simulink library "dynamics_lib"  (R2023b)
settings: Solver=VariableStepAuto  StartTime=0.0  StopTime=10.0  RelTol=1e-3
libraries: Raptor_lib x129, cstblocks x1, autolibshared x1
(part 2 of 2)

== system dynamics_lib/vehicleModel ==
  Constant : Constant  Value=5
  Constant1 : Constant  Value=5
  Display : Display
  Scope : Scope  NumInputPorts=6
  Vehicle Body 3DOF Single Track : autolibshared/Vehicle Body 3DOF Single Track  trackMode=Single (bicycle)  inputMode=External longitudinal velocity  frontSteerMode=on  rearSteerMode=off  windMode=off  muMode=off  extFMode=off  extMMode=off  htchFMode=off  htchMMode=off  extXo=off  extpsio=off  extxdoto=off  extro=off  extYo=off  extTamb=off  extydoto=off  aMode=2  NF=2  NR=2  m=272.16  a=0.76835  b=0.76835  h=0.31612  dh=1  hh=0.2  X_o=0  xdot_o=0  CalphaMode=off  sigmaMode=off  d=0  hl=0  w=[1.4,1.4]  Cy_f=18550.11  Cy_r=18550.11  sigma_f=.1  sigma_r=.1  alpha_f_brk=[-.1 .1]  Cy_f_data=[-9e3 9e3]  alpha_r_brk=[-.1 .1]  Cy_r_data=[-9e3 9e3]  Y_o=0  ydot_o=0  Izz=113.95  psi_o=0  r_o=0  Af=1.207  Cd=.3  Cl=.1  Cpm=.1  beta_w=[0 0.01:0.01:0.3]  Cs=[0 0.01:0.01:0.3]  Cym=[0 1e-6:0.01:0.3]  Pabs=101325  Tair=273  g=9.81  mu=1  xdot_tol=.01  Fznom=5000  Fxtire_sat=7e4  Fytire_sat=7e4  longOff=0  latOff=0  vertOff=0  wrapAng=off
  wires:
  Vehicle Body 3DOF Single Track/1 -> Display/1
  Vehicle Body 3DOF Single Track/2 -> Scope/1
  Vehicle Body 3DOF Single Track/3 -> Scope/2
  Vehicle Body 3DOF Single Track/4 -> Scope/3
  Vehicle Body 3DOF Single Track/5 -> Scope/4
  Vehicle Body 3DOF Single Track/6 -> Scope/5
  Vehicle Body 3DOF Single Track/7 -> Scope/6
  Constant/1 -> Vehicle Body 3DOF Single Track/2
  Constant1/1 -> Vehicle Body 3DOF Single Track/1

== matlab function dynamics_lib/rearNSMWT/rearNSMWT ==
  data: rearNonSuspendedMass input; rearNSMWT output; MM5_ay input; rearNonSuspendedMassCGHeight input; rearTrack input
function rearNSMWT = fcn(rearNonSuspendedMass, MM5_ay, ...
    rearNonSuspendedMassCGHeight, rearTrack)

rearNSMWT = rearNonSuspendedMass*2*MM5_ay*...
    rearNonSuspendedMassCGHeight/rearTrack;

== matlab function dynamics_lib/frontGeoWT/frontGeoWT ==
  data: suspendedMass input; frontGeoWT output; suspendedMassWeightDistribution input; MM5_ay input; frontRollCenterHeight input; frontTrack input
function frontGeoWT = fcn(suspendedMass, ...
    suspendedMassWeightDistribution, MM5_ay, frontRollCenterHeight, ...
        frontTrack)

frontGeoWT = suspendedMass*(suspendedMassWeightDistribution/100)*MM5_ay*...
    frontRollCenterHeight/frontTrack;

== matlab function dynamics_lib/rearGeoWT/rearGeoWT ==
  data: suspendedMass input; rearGeoWT output; suspendedMassWeightDistribution input; MM5_ay input; rearRollCenterHeight input; rearTrack input
function rearGeoWT = fcn(suspendedMass, ...
    suspendedMassWeightDistribution, MM5_ay, rearRollCenterHeight, ...
        rearTrack)

rearGeoWT = (suspendedMass*((100-suspendedMassWeightDistribution)/100))*...
    MM5_ay*rearRollCenterHeight/rearTrack;

== matlab function dynamics_lib/antiRollFrontSprings/antiRollFrontSprings ==
  data: frontTrack input; antiRollFrontSprings output; frontWheelRate input
function antiRollFrontSprings = fcn(frontTrack, frontWheelRate)

antiRollFrontSprings = ((frontTrack/1000)^2*tan(1)* ...
    (frontWheelRate*1000))/2;

== matlab function dynamics_lib/antiRollRearSprings/antiRollRearSprings ==
  data: rearTrack input; antiRollRearSprings output; rearWheelRate input
function antiRollRearSprings = fcn(rearTrack, rearWheelRate)

antiRollRearSprings = ((rearTrack/1000)^2*tan(1)* ...
    (rearWheelRate*1000))/2;

== matlab function dynamics_lib/frontWheelRate/frontWheelRate ==
  data: frontSpringStiffness input; frontWheelRate output; frontSpringMotionRatio input
function frontWheelRate = fcn(frontSpringStiffness, frontSpringMotionRatio)

frontWheelRate = frontSpringStiffness/frontSpringMotionRatio^2;

== matlab function dynamics_lib/antiRollFrontAxleAndTire/antiRollFrontAxleAndTire ==
  data: antiRollFrontAxleAndTire output; antiRollFrontSprings input; antiRollFrontARB input; antiRollFrontTires input
function antiRollFrontAxleAndTire = fcn(antiRollFrontSprings, ...
    antiRollFrontARB, antiRollFrontTires)

antiRollFrontAxleAndTire = ((antiRollFrontSprings+antiRollFrontARB)* ...
    antiRollFrontTires)/((antiRollFrontSprings+antiRollFrontARB)+ ...
        antiRollFrontTires);

== matlab function dynamics_lib/antiRollRearAxleAndTire/antiRollRearAxleAndTire ==
  data: antiRollRearAxleAndTire output; antiRollRearSprings input; antiRollRearARB input; antiRollRearTires input
function antiRollRearAxleAndTire = fcn(antiRollRearSprings, ...
    antiRollRearARB, antiRollRearTires)

antiRollRearAxleAndTire = ((antiRollRearSprings+antiRollRearARB)* ...
    antiRollRearTires)/((antiRollRearSprings+antiRollRearARB)+ ...
        antiRollRearTires);

== matlab function dynamics_lib/antiRollTotal/antiRollTotal ==
  data: antiRollFrontAxleAndTire input; antiRollTotal output; antiRollRearAxleAndTire input
function antiRollTotal = fcn(antiRollFrontAxleAndTire, ...
    antiRollRearAxleAndTire)

antiRollTotal = antiRollFrontAxleAndTire+antiRollRearAxleAndTire;

== matlab function dynamics_lib/frontElWT/frontElWT ==
  data: frontElWT output; suspendedMass input; MM5_ay input; deltaZ input; antiRollFrontAxleAndTire input; antiRollTotal input; frontTrack input
function frontElWT = fcn(suspendedMass, MM5_ay, deltaZ, ...
    antiRollFrontAxleAndTire, antiRollTotal, frontTrack)

frontElWT = (suspendedMass*MM5_ay*deltaZ* ...
    (antiRollFrontAxleAndTire/antiRollTotal))/frontTrack;

== matlab function dynamics_lib/rearElWT/rearElWT ==
  data: rearElWT output; suspendedMass input; MM5_ay input; deltaZ input; antiRollRearAxleAndTire input; antiRollTotal input; rearTrack input
function rearElWT = fcn(suspendedMass, MM5_ay, deltaZ, ...
    antiRollRearAxleAndTire, antiRollTotal, rearTrack)

rearElWT = (suspendedMass*MM5_ay*deltaZ* ...
    (antiRollRearAxleAndTire/antiRollTotal))/rearTrack;

== matlab function dynamics_lib/frontTotalWT/frontTotalWT ==
  data: frontNSMWT input; frontTotalWT output; frontElWT input; frontGeoWT input
function frontTotalWT = fcn(frontNSMWT, frontElWT, frontGeoWT)

frontTotalWT = frontNSMWT+frontElWT+frontGeoWT;

== matlab function dynamics_lib/rearTotalWT/rearTotalWT ==
  data: rearNSMWT input; rearTotalWT output; rearElWT input; rearGeoWT input
function rearTotalWT = fcn(rearNSMWT, rearElWT, rearGeoWT)

rearTotalWT = rearNSMWT+rearElWT+rearGeoWT;

== matlab function dynamics_lib/dynamicLoadFL/dynamicLoadFL ==
  data: dynamicLoadFL output; totalMass input; totalMassDistribution input; totalDownForce input; downForceDistribution input; totalFrontWT input; gravity input
function dynamicLoadFL = fcn(totalMass, totalMassDistribution, ...
    totalDownForce, downForceDistribution, totalFrontWT, gravity)

dynamicLoadFL = (totalMass*totalMassDistribution/100*0.5+totalDownForce*...
    downForceDistribution/100/2-totalFrontWT)*gravity;

== matlab function dynamics_lib/dynamicLoadFR/dynamicLoadFR ==
  data: dynamicLoadFR output; totalMass input; totalMassDistribution input; totalDownForce input; downForceDistribution input; totalFrontWT input; gravity input
function dynamicLoadFR = fcn(totalMass, totalMassDistribution, ...
    totalDownForce, downForceDistribution, totalFrontWT, gravity)

dynamicLoadFR = (totalMass*totalMassDistribution/100*0.5+totalDownForce*...
    downForceDistribution/100/2+totalFrontWT)*gravity;

== matlab function dynamics_lib/dynamicLoadRL/dynamicLoadRL ==
  data: dynamicLoadRL output; totalMass input; totalMassDistribution input; totalDownForce input; downForceDistribution input; totalRearWT input; gravity input
function dynamicLoadRL = fcn(totalMass, totalMassDistribution, ...
    totalDownForce, downForceDistribution, totalRearWT, gravity)

dynamicLoadRL = (totalMass*(100-totalMassDistribution)/100*0.5+ ...
    totalDownForce*(100-downForceDistribution)/100/2-totalRearWT)*gravity;

== matlab function dynamics_lib/dynamicLoadRR/dynamicLoadRR ==
  data: dynamicLoadRR output; totalMass input; totalMassDistribution input; totalDownForce input; downForceDistribution input; totalRearWT input; gravity input
function dynamicLoadRR = fcn(totalMass, totalMassDistribution, ...
    totalDownForce, downForceDistribution, totalRearWT, gravity)

dynamicLoadRR = (totalMass*(100-totalMassDistribution)/100*0.5+ ...
    totalDownForce*(100-downForceDistribution)/100/2+totalRearWT)*gravity;

== matlab function dynamics_lib/fz/fz ==
  data: frontSpringStiffness input; dynamicLoadFL output; frontSpringMotionRatio input; rearSpringStiffness input; rearSpringMotionRatio input; frontNonSuspendedMass input; MM5_ay input; frontNonSuspendedMassCGHeight input; frontTrack input; suspendedMass input; suspendedMassWeightDistribution input; frontRollCenterHeight input; frontTireStiffness input; frontARBStiffness input; frontARBMotionRatio input; rearTrack input; rearARBStiffness input; rearARBMotionRatio input; rearTireStiffness input; rearNonSuspendedMass input; rearNonSuspendedMassCGHeight input; rearRollCenterHeight input; suspendedMassCGCoordinatesZ input; wheelBase input; totalMass input; totalMassDistribution input; totalDownForce input; downForceDistribution input; gravity input; dynamicLoadFR output; dynamicLoadRL output; dynamicLoadRR output
function [dynamicLoadFL, dynamicLoadFR, dynamicLoadRL, dynamicLoadRR] = ...
    fz(frontSpringStiffness, frontSpringMotionRatio, ...
    rearSpringStiffness, rearSpringMotionRatio, frontNonSuspendedMass, ...
    MM5_ay, frontNonSuspendedMassCGHeight, frontTrack, suspendedMass, ...
    suspendedMassWeightDistribution, frontRollCenterHeight, ...
    frontTireStiffness, frontARBStiffness, frontARBMotionRatio, ...
    rearTrack, rearARBStiffness, rearARBMotionRatio, ...
    rearTireStiffness, rearNonSuspendedMass, ...
    rearNonSuspendedMassCGHeight, rearRollCenterHeight, ...
    suspendedMassCGCoordinatesZ, wheelBase, totalMass, ...
    totalMassDistribution, totalDownForce, downForceDistribution, gravity)



frontWheelRate = frontSpringStiffness/frontSpringMotionRatio^2;
rearWheelRate = rearSpringStiffness/rearSpringMotionRatio^2;
frontNSMWT = frontNonSuspendedMass*2*MM5_ay*...
    frontNonSuspendedMassCGHeight/frontTrack;
frontGeoWT = suspendedMass*(suspendedMassWeightDistribution/100)*MM5_ay*...
    frontRollCenterHeight/frontTrack;
antiRollFrontTires = ((frontTrack/1000)^2*tan(1)*frontTireStiffness* ...
    1000)/2;
antiRollFrontARB = (frontARBStiffness*1000*(frontTrack/1000)^2*tan(1))/...
    frontARBMotionRatio^2;
antiRollFrontSprings = ((frontTrack/1000)^2*tan(1)* ...
    (frontWheelRate*1000))/2;
antiRollRearSprings = ((rearTrack/1000)^2*tan(1)* ...
    (rearWheelRate*1000))/2;
antiRollRearARB = (rearARBStiffness*1000*(rearTrack/1000)^2*tan(1))/...
    rearARBMotionRatio^2;
antiRollRearTires = ((rearTrack/1000)^2*tan(1)*rearTireStiffness* ...
    1000)/2;
rearNSMWT = rearNonSuspendedMass*2*MM5_ay*...
    rearNonSuspendedMassCGHeight/rearTrack;
rearGeoWT = (suspendedMass*((100-suspendedMassWeightDistribution)/100))*...
    MM5_ay*rearRollCenterHeight/rearTrack;
deltaZ = suspendedMassCGCoordinatesZ-...
    (((rearRollCenterHeight-frontRollCenterHeight)/wheelBase* ...
        ((100-suspendedMassWeightDistribution)/100*wheelBase))+ ...
            frontRollCenterHeight);
antiRollFrontAxleAndTire = ((antiRollFrontSprings+antiRollFrontARB)* ...
    antiRollFrontTires)/((antiRollFrontSprings+antiRollFrontARB)+ ...
        antiRollFrontTires);
antiRollRearAxleAndTire = ((antiRollRearSprings+antiRollRearARB)* ...
    antiRollRearTires)/((antiRollRearSprings+antiRollRearARB)+ ...
        antiRollRearTires);
antiRollTotal = antiRollFrontAxleAndTire+antiRollRearAxleAndTire;
frontElWT = (suspendedMass*MM5_ay*deltaZ* ...
    (antiRollFrontAxleAndTire/antiRollTotal))/frontTrack;
rearElWT = (suspendedMass*MM5_ay*deltaZ* ...
    (antiRollRearAxleAndTire/antiRollTotal))/rearTrack;
frontTotalWT = frontNSMWT+frontElWT+frontGeoWT;
rearTotalWT = rearNSMWT+rearElWT+rearGeoWT;
dynamicLoadFL = (totalMass*totalMassDistribution/100*0.5+totalDownForce*...
    downForceDistribution/100/2-frontTotalWT)*gravity;
dynamicLoadFR = (totalMass*totalMassDistribution/100*0.5+totalDownForce*...
    downForceDistribution/100/2+frontTotalWT)*gravity;
dynamicLoadRL = (totalMass*(100-totalMassDistribution)/100*0.5+ ...
    totalDownForce*(100-downForceDistribution)/100/2-rearTotalWT)*gravity;
dynamicLoadRR = (totalMass*(100-totalMassDistribution)/100*0.5+ ...
    totalDownForce*(100-downForceDistribution)/100/2+rearTotalWT)*gravity;

== matlab function dynamics_lib/corneringStiffness/MATLAB Function ==
  data: Fz input; Ca output; pressure input; inclangl input; FNOMIN input; LFZO input; NOMPRES input; LCY input; PCY1 input; PDY1 input; PDY2 input; PPY3 input; PPY4 input; PDY3 input; LMUY input; PKY1 input; PPY1 input; PKY3 input; PKY4 input; PKY2 input; PKY5 input; PPY2 input; LKY input; ZETA2 input; ZETA3 input
function Ca = fcn(Fz,pressure,inclangl,FNOMIN,LFZO,NOMPRES,LCY,PCY1, ...
    PDY1,PDY2,PPY3,PPY4,PDY3,LMUY,PKY1,PPY1,PKY3,PKY4,PKY2,PKY5,PPY2, ...
    LKY,ZETA2,ZETA3)

gammaAst = sin(inclangl);
gammaAst2 = gammaAst.^2;

Fz0_ = FNOMIN.*LFZO;

dfz = (Fz-Fz0_)./Fz0_;
 
pi0 = NOMPRES;
dpi = (pressure-pi0)./pi0;
dpi2 = dpi.^2;

Cy = LCY.*PCY1;

muy = (PDY1+PDY2.*dfz).*(1+PPY3.*dpi+PPY4.*dpi2)...
    .*(1-PDY3.*gammaAst2).*LMUY;

Dy = muy.*Fz.*ZETA2;

Kya = PKY1.*Fz0_...
    .*(1+PPY1.*dpi)...
    .*(1-PKY3.*abs(gammaAst))...
    .*sin(PKY4.*atan(Fz./Fz0_./((PKY2+PKY5.*gammaAst2)...
    .*(1+PPY2.*dpi)))).*LKY.*ZETA3;

signCy = sign(Cy);
signCy(~signCy) = 1;
By = Kya./(Cy.*Dy + eps(Cy).*signCy);

Ca = -(By*Cy*Dy);

== matlab function dynamics_lib/longitudinalStiffness/MATLAB Function ==
  data: Fz input; Cx output; pressure input; inclangl input; FNOMIN input; LFZO input; NOMPRES input; PCX1 input; LCX input; LMUX input; PDX1 input; PDX2 input; PPX3 input; PPX4 input; PDX3 input; ZETA1 input; LKX input; PKX1 input; PKX2 input; PKX3 input; PPX1 input; PPX2 input
function Cx = fcn(Fz,pressure,inclangl,FNOMIN,LFZO,NOMPRES,PCX1,LCX, ...
    LMUX,PDX1,PDX2,PPX3,PPX4,PDX3,ZETA1,LKX,PKX1,PKX2,PKX3,PPX1,PPX2)

Fz0_ = FNOMIN.*LFZO;
dfz = (Fz-Fz0_)./Fz0_;
 
pi0 = NOMPRES;
dpi = (pressure-pi0)./pi0;

Cx = PCX1.*LCX;

mux = LMUX.*(PDX1+PDX2.*dfz).*(1+PPX3.*dpi+PPX4.*dpi.^2).*(1-PDX3.*inclangl.^2);

Dx = mux.*Fz*ZETA1;

Kxk = LKX.*Fz.*(PKX1+PKX2.*dfz).*exp(PKX3.*dfz).*(1+PPX1.*dpi+PPX2.*dpi.^2);

Bx = Kxk./(Cx.*Dx+eps(Kxk));

Cx = Bx*Cx*Dx;

== matlab function dynamics_lib/lateralDynamics/A ==
  data: Cf_rad input; A output; Cr_rad input; totalMass input; vx input; a input; b input; d input; Iz input; Re input; J input; Ckfl input; Ckfr input; Ckrl input; Ckrr input; x3 input; x4 input; x5 input; x6 input
function A = fcn(Cf_rad,Cr_rad,totalMass,vx,a,b,d,Iz,Re,J,Ckfl,Ckfr,Ckrl,Ckrr,x3,x4,x5,x6)

A = [-(2*Cf_rad - 2*Cr_rad)/(totalMass*vx), - ((2*Cf_rad*a)/vx + (2*Cr_rad*b)/vx)/(totalMass*vx) - 1,                                                                             0,                                                                             0,                                                                             0,                                                                             0; ...
        -(2*Cf_rad*a - 2*Cr_rad*b)/Iz,              -((2*Cf_rad*a^2)/vx + (2*Cr_rad*b^2)/vx)/Iz,                                                              -(Ckfl*d)/(2*Iz),                                                               (Ckfr*d)/(2*Iz),                                                              -(Ckrl*d)/(2*Iz),                                                               (Ckrr*d)/(2*Iz); ...
                                    0,                                                        0, - Ckfl*(Re^2/(J*vx) + (4*x3 + 4)/(totalMass*vx)) - (4*Ckfl*x3)/(totalMass*vx),                                                                             0,                                                                             0,                                                                             0; ...
                                    0,                                                        0,                                                                             0, - Ckfr*(Re^2/(J*vx) + (4*x4 + 4)/(totalMass*vx)) - (4*Ckfr*x4)/(totalMass*vx),                                                                             0,                                                                             0; ...
                                    0,                                                        0,                                                                             0,                                                                             0, - Ckrl*(Re^2/(J*vx) + (4*x5 + 4)/(totalMass*vx)) - (4*Ckrl*x5)/(totalMass*vx),                                                                             0; ...
                                    0,                                                        0,                                                                             0,                                                                             0,                                                                             0, - Ckrr*(Re^2/(J*vx) + (4*x6 + 4)/(totalMass*vx)) - (4*Ckrr*x6)/(totalMass*vx)];

== matlab function dynamics_lib/deltaZ/deltaZ ==
  data: wheelBase input; deltaZ output; suspendedMassWeightDistribution input; suspendedMassCGCoordinatesZ input; frontRollCenterHeight input; rearRollCenterHeight input
function deltaZ = fcn(wheelBase, suspendedMassWeightDistribution, ...
    suspendedMassCGCoordinatesZ, frontRollCenterHeight, ...
        rearRollCenterHeight)

deltaZ = suspendedMassCGCoordinatesZ-...
    (((rearRollCenterHeight-frontRollCenterHeight)/wheelBase* ...
        ((100-suspendedMassWeightDistribution)/100*wheelBase))+ ...
            frontRollCenterHeight);

== matlab function dynamics_lib/lateralDynamics/MATLAB Function1 ==
  data: vx input; x3 output; w1 input; Re input
function x3 = fcn(vx,w1,Re)

x3=-(vx-w1*Re)/vx;

== matlab function dynamics_lib/lateralDynamics/MATLAB Function2 ==
  data: vx input; x4 output; w2 input; Re input
function x4 = fcn(vx,w2,Re)

x4=-(vx-w2*Re)/vx;

== matlab function dynamics_lib/lateralDynamics/MATLAB Function3 ==
  data: vx input; x5 output; w3 input; Re input
function x5 = fcn(vx,w3,Re)

x5=-(vx-w3*Re)/vx;

== matlab function dynamics_lib/lateralDynamics/MATLAB Function4 ==
  data: vx input; x6 output; w4 input; Re input
function x6 = fcn(vx,w4,Re)

x6=-(vx-w4*Re)/vx;

== matlab function dynamics_lib/lateralDynamics/B ==
  data: Re input; B output; J input; vx input
function B = fcn(Re,J,vx)

B = [ 0 0 0 0; ...
    0 0 0 0; ...
    Re/(J*vx),         0,         0,         0; ...
        0, Re/(J*vx),         0,         0; ...
        0,         0, Re/(J*vx),         0; ...
        0,         0,         0, Re/(J*vx)];

== matlab function dynamics_lib/longitudinalSlipEstimator/s ==
  data: wheelCenterSpeedFL input; sfl output; wheelCenterSpeedFR input; wheelCenterSpeedRL input; wheelCenterSpeedRR input; wheelRadius input; angularSpeedFL input; angularSpeedFR input; angularSpeedRL input; angularSpeedRR input; sfr output; srl output; srr output
function [sfl,sfr,srl,srr] = fcn(wheelCenterSpeedFL, ...
    wheelCenterSpeedFR,wheelCenterSpeedRL,wheelCenterSpeedRR, ...
    wheelRadius,angularSpeedFL,angularSpeedFR,angularSpeedRL, ...
    angularSpeedRR)
% longslip = -(Vwheelcenter-Rwheelradius*R/sangularspeed)/Vwheelcenter
% full wheel lockup is -1
% full wheel slip is 1
% free rolling is 0
sfl = -(wheelCenterSpeedFL-wheelRadius* ...
    angularSpeedFL)/(wheelCenterSpeedFL);
sfr = -(wheelCenterSpeedFR-wheelRadius* ...
    angularSpeedFR)/(wheelCenterSpeedFR);
srl = -(wheelCenterSpeedRL-wheelRadius* ...
    angularSpeedRL)/(wheelCenterSpeedRL);
srr = -(wheelCenterSpeedRR-wheelRadius* ...
    angularSpeedRR)/(wheelCenterSpeedRR);

== matlab function dynamics_lib/slipAngleEstimator/a ==
  data: lateralVelocity input; afl output; yawRate input; frontWheelBase input; rearWheelBase input; wheelCenterSpeedFL input; wheelCenterSpeedFR input; wheelCenterSpeedRL input; wheelCenterSpeedRR input; frontTrack input; rearTrack input; steeringAngle input; afr output; arl output; arr output
function [afl,afr,arl,arr] = fcn(lateralVelocity,yawRate, ...
    frontWheelBase,rearWheelBase,wheelCenterSpeedFL, ...
    wheelCenterSpeedFR,wheelCenterSpeedRL,wheelCenterSpeedRR, ...
    frontTrack,rearTrack,steeringAngle)

afl = (lateralVelocity+yawRate*frontWheelBase)/(wheelCenterSpeedFL+ ...
    yawRate*frontTrack/2)-steeringAngle;
afr = (lateralVelocity+yawRate*frontWheelBase)/(wheelCenterSpeedFR- ...
    yawRate*frontTrack/2)-steeringAngle;
arl = (lateralVelocity-yawRate*rearWheelBase)/(wheelCenterSpeedRL- ...
    yawRate*rearTrack/2);
arr = (lateralVelocity-yawRate*rearWheelBase)/(wheelCenterSpeedRR+ ...
    yawRate*rearTrack/2);

== matlab function dynamics_lib/rearWheelRate/rearWheelRate ==
  data: rearSpringStiffness input; rearWheelRate output; rearSpringMotionRatio input
function rearWheelRate = fcn(rearSpringStiffness, rearSpringMotionRatio)

rearWheelRate = rearSpringStiffness/rearSpringMotionRatio^2;

== matlab function dynamics_lib/antiRollFrontARB/antiRollFrontARB ==
  data: frontARBStiffness input; antiRollFrontARB output; frontTrack input; frontARBMotionRatio input
function antiRollFrontARB = fcn(frontARBStiffness, frontTrack, ...
    frontARBMotionRatio)

antiRollFrontARB = (frontARBStiffness*1000*(frontTrack/1000)^2*tan(1))/...
    frontARBMotionRatio^2;

== matlab function dynamics_lib/antiRollRearARB/antiRollRearARB ==
  data: rearARBStiffness input; antiRollRearARB output; rearTrack input; rearARBMotionRatio input
function antiRollRearARB = fcn(rearARBStiffness, rearTrack, ...
    rearARBMotionRatio)

antiRollRearARB = (rearARBStiffness*1000*(rearTrack/1000)^2*tan(1))/...
    rearARBMotionRatio^2;

== matlab function dynamics_lib/antiRollFrontTires/antiRollFrontTires ==
  data: frontTrack input; antiRollFrontTires output; frontTireStiffness input
function antiRollFrontTires = fcn(frontTrack, frontTireStiffness)

antiRollFrontTires = ((frontTrack/1000)^2*tan(1)*frontTireStiffness* ...
    1000)/2;

== matlab function dynamics_lib/antiRollRearTires/antiRollRearTires ==
  data: rearTrack input; antiRollRearTires output; rearTireStiffness input
function antiRollRearTires = fcn(rearTrack, rearTireStiffness)

antiRollRearTires = ((rearTrack/1000)^2*tan(1)*rearTireStiffness* ...
    1000)/2;

== matlab function dynamics_lib/frontNSMWT/frontNSMWT ==
  data: frontNonSuspendedMass input; frontNSMWT output; MM5_ay input; frontNonSuspendedMassCGHeight input; frontTrack input
function frontNSMWT = fcn(frontNonSuspendedMass, MM5_ay, ...
    frontNonSuspendedMassCGHeight, frontTrack)

frontNSMWT = frontNonSuspendedMass*2*MM5_ay*...
    frontNonSuspendedMassCGHeight/frontTrack;
